simulink model "enforce_constraint"  (R2021b)
settings: Solver=FixedStepDiscrete  StartTime=0.0  StopTime=10.0  FixedStep=info_.slx_sample_time_for_con_enf  RelTol=1e-3
undefined symbols (not defined in the file): agent_act_number, agent_obs_number, slx_constr_bound, slx_max_t, slx_min_t
libraries: dspindex x2
settings Model: Creator=krzysztof  LastModifiedBy=krzysztof
settings DataIOCC: SignalLogging=off

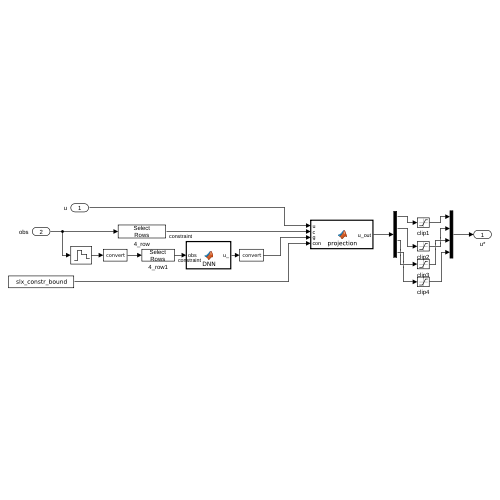
[thumbnail: Simulink's stored preview of the top-level diagram]
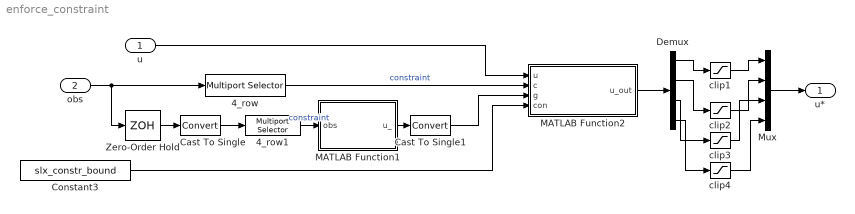
== system enforce_constraint ==
  u : Inport  PortDimensions=[agent_act_number 1]
  obs : Inport  Port=2  PortDimensions=[agent_obs_number 1]
  4_row : dspindex/Multiport Selector  rowsOrCols=Rows  idxCellArray={4}  idxErrMode=Clip Index
  4_row1 : dspindex/Multiport Selector  rowsOrCols=Rows  idxCellArray={1:4}  idxErrMode=Clip Index
  Cast To Single : DataTypeConversion
  Cast To Single1 : DataTypeConversion
  Constant3 : Constant  Value=slx_constr_bound
  Demux : Demux
  MATLAB Function1 : MATLAB Function  TreatAsAtomicUnit=on
  MATLAB Function2 : MATLAB Function  TreatAsAtomicUnit=on
  Mux : Mux
  Zero-Order Hold : ZeroOrderHold  SampleTime=-1
  clip{1..4} (4 alike) : Saturate  UpperLimit=slx_max_t  LowerLimit=slx_min_t
  u* : Outport
  wires:
  Zero-Order Hold/1 -> Cast To Single/1
  Cast To Single/1 -> 4_row1/1
  4_row/1 -> MATLAB Function2/2(c)  "constraint"
  u/1 -> MATLAB Function2/1(u)
  Constant3/1 -> MATLAB Function2/4(con)
  Mux/1 -> u*/1
  MATLAB Function2/1(u_out) -> Demux/1
  Demux/1 -> clip1/1
  clip1/1 -> Mux/1
  Demux/2 -> clip2/1
  clip2/1 -> Mux/2
  obs/1 -> 4_row/1, Zero-Order Hold/1
  Cast To Single1/1 -> MATLAB Function2/3(g)
  MATLAB Function1/1(u_) -> Cast To Single1/1
  4_row1/1 -> MATLAB Function1/1(obs)  "constraint"
  Demux/3 -> clip3/1
  clip3/1 -> Mux/3
  Demux/4 -> clip4/1
  clip4/1 -> Mux/4

== matlab function enforce_constraint/MATLAB Function2 ==
  data: u input; c input; g input; u_out output; con input
function u_out = projection(u,c,g,con)
c = c - con; % c - Ci <= 0
coder.extrinsic('projection_func')
 u_ = double([0; 0; 0]);
u_ = double(projection_func(g,c,u))';

%% temporal fix
u_out = u_(1:4);

== matlab function enforce_constraint/MATLAB Function1 ==
  data: obs input; u_ output
function u_ = DNN(obs)
    coder.extrinsic('predict_with_NN')
    % obs - four variable vector
    u_ = single([0; 0; 0]);
    u_ = predict_with_NN(obs);
end
